simulink model "Final"  (R2018b)
settings: Solver=FixedStepAuto  StartTime=0.0  StopTime=300  RelTol=1e-3  EnableMultiTasking=on
libraries: arduinolib x4, LCDlib x1, arduinosensorlib x1
settings Model: SimulationMode=external  ExtModeTrigDuration=2  Creator=Pruthvi Gabani  LastModifiedBy=Pruthvi Gabani
settings OptimizationCC: EnhancedBackFolding=on  PassReuseOutputArgsAs=Individual arguments  MaxStackSize=64  OptimizeBlockOrder=speed  DifferentSizesBufferReuse=on  OptimizationCustomize=off
settings DebuggingCC: ParameterTunabilityLossMsg=error
settings HardwareCC: ProdBitPerInt=16  ProdBitPerPointer=16  ProdBitPerSizeT=16  ProdBitPerPtrDiffT=16  ProdLargestAtomicFloat=None  ProdWordSize=8  ProdHWDeviceType=Atmel->AVR
settings SFSimCC: MATLABDynamicMemAlloc=off
settings RTWCC: SystemTargetFile=ert.tlc  HardwareBoard=Arduino Uno  TemplateMakefile=ert_default_tmf  GenerateReport=on  Toolchain=Arduino AVR  BuildConfiguration=Faster Runs  IncludeHyperlinkInReport=on  LaunchReport=on  GenerateTraceInfo=on  GenerateTraceReport=on  GenerateTraceReportSl=on  GenerateTraceReportSf=on  GenerateTraceReportEml=on
settings CodeAppCC: ForceParamTrailComments=on  IgnoreCustomStorageClasses=off  OperatorAnnotations=on  SimulinkDataObjDesc=on  SFDataObjDesc=on  InsertBlockDesc=on
settings ERTTargetCC: SupportContinuousTime=on  SupportVariableSizeSignals=on

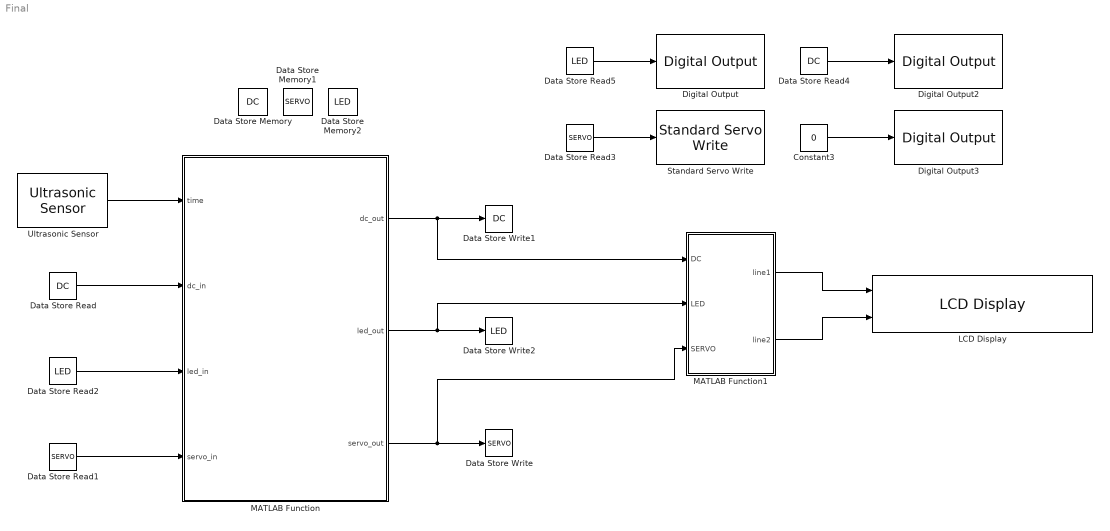
== system Final ==
  Constant3 : Constant  Value=0  SampleTime=-1
  Data Store Memory : DataStoreMemory  DataStoreName=DC  ReadBeforeWriteMsg=warning  WriteAfterWriteMsg=warning  WriteAfterReadMsg=warning  ShowAdditionalParam=off
  Data Store Memory1 : DataStoreMemory  DataStoreName=SERVO  ReadBeforeWriteMsg=warning  WriteAfterWriteMsg=warning  WriteAfterReadMsg=warning  ShowAdditionalParam=off
  Data Store Memory2 : DataStoreMemory  DataStoreName=LED  ReadBeforeWriteMsg=warning  WriteAfterWriteMsg=warning  WriteAfterReadMsg=warning  ShowAdditionalParam=off
  Data Store Read : DataStoreRead  DataStoreName=DC
  Data Store Read1 : DataStoreRead  DataStoreName=SERVO
  Data Store Read2 : DataStoreRead  DataStoreName=LED
  Data Store Read3 : DataStoreRead  DataStoreName=SERVO
  Data Store Read4 : DataStoreRead  DataStoreName=DC
  Data Store Read5 : DataStoreRead  DataStoreName=LED
  Data Store Write : DataStoreWrite  DataStoreName=SERVO
  Data Store Write1 : DataStoreWrite  DataStoreName=DC
  Data Store Write2 : DataStoreWrite  DataStoreName=LED
  Digital Output : arduinolib/Digital Output  pinNumber=13  blockPlatform=arduino
  Digital Output2 : arduinolib/Digital Output  pinNumber=6  blockPlatform=arduino
  Digital Output3 : arduinolib/Digital Output  pinNumber=7  blockPlatform=arduino
  LCD Display : LCDlib/LCD Display  pins=[10,9,5,4,3,2]
      settings: SourceProductName=LCD Library
  MATLAB Function : MATLAB Function  TreatAsAtomicUnit=on
  MATLAB Function1 : MATLAB Function  TreatAsAtomicUnit=on
  Standard Servo Write : arduinolib/Standard Servo Write  pinNumber=8  ServoIndex=0  blockPlatform=ARDUINO
      settings: SourceProductName=Simulink Support Package for Arduino Hardware
  Ultrasonic Sensor : arduinosensorlib/Ultrasonic Sensor  NumSignalPins=2  TrigPin=11  EchoPin=12  SignalPin=3  SampleTime_=1  blockPlatform=ARDUINO
      settings: SourceProductName=Simulink Support Package for Arduino Hardware
  wires:
  Data Store Read5/1 -> Digital Output/1
  Data Store Read/1 -> MATLAB Function/2(dc_in)
  Data Store Read3/1 -> Standard Servo Write/1
  Data Store Read1/1 -> MATLAB Function/4(servo_in)
  Data Store Read4/1 -> Digital Output2/1
  Constant3/1 -> Digital Output3/1
  Data Store Read2/1 -> MATLAB Function/3(led_in)
  MATLAB Function/1(dc_out) -> Data Store Write1/1, MATLAB Function1/1(DC)
  MATLAB Function/2(led_out) -> MATLAB Function1/2(LED), Data Store Write2/1
  MATLAB Function/3(servo_out) -> MATLAB Function1/3(SERVO), Data Store Write/1
  MATLAB Function1/1(line1) -> LCD Display/1
  MATLAB Function1/2(line2) -> LCD Display/2
  Ultrasonic Sensor/1 -> MATLAB Function/1(time)

== matlab function Final/MATLAB Function1 ==
  data: DC input; line1 output; LED input; SERVO input; line2 output
function [line1,line2] = fcn(DC,LED,SERVO)
 if DC == 1
     line1=[[68],[67],[32],[77],[111],[116],[111],[114],[32],[82],[80],[77],[58]];
 elseif LED == 1
    line1 = [[65],[76],[69],[82],[84],[33],[32],[32],[32],[32],[32],[32],[32]];
else 
    line1 = [[32],[32],[32],[32],[32],[32],[32],[32],[32],[32],[32],[32],[32]];
end
if SERVO == 180
    line2= [[84],[85],[82],[78],[32],[76],[69],[70],[84],[32],[32]];
elseif SERVO == 0
    line2= [[84],[85],[82],[78],[32],[82],[73],[71],[72],[84],[32]];
elseif DC == 1
    line2 = [[49],[56],[50],[57],[32],[32],[32],[32],[32],[32],[32]];
else 
    line2= [[32],[32],[32],[32],[32],[32],[32],[32],[32],[32],[32]];
end 
end

== matlab function Final/MATLAB Function ==
  data: dc_out output; led_out output; time input; servo_out output; dc_in input; led_in input; servo_in input
function [dc_out,led_out,servo_out]  = MainCOde(time,dc_in,led_in, servo_in)
distance = (time*343)/2;

if distance > 40
    servo_out = 90;
    dc_out=1;
    led_out = 0;
elseif distance > 0 && distance < 15
    servo_out = 180;
    dc_out  = 0;
    led_out=1;
elseif distance > 15 && distance < 30
    servo_out = 0;
    dc_out  = 0;
    led_out=1;
else
    servo_out = servo_in;
    dc_out= dc_in;
    led_out=led_in;
end
end
